simulink model "simulator_LQR"  (R2018b)
settings: Solver=VariableStepAuto  StartTime=0.0  StopTime=150  RelTol=1e-5
values from neighbouring files (symbols this model uses):
  C = [1 0 0;0 1 0; 0 0 1]    [parameters_LQR.m]
  LQR_fast = [830.7,	3032.2,	1268.5]    [parameters_LQR.m]
  LQR_slow = [624.5,	2682.3,	1569.3]    [parameters_LQR.m]
  Nbar = Nu + [(LQR_slow(2)+LQR_fast(2))/2 (LQR_slow(3)+LQR_fast(3))/2]*Nx    [parameters_LQR.m]
undefined symbols (not defined in the file or in its folder): A, B
libraries: simulink_extras x2
settings Model: Creator=jenny  LastModifiedBy=jenny

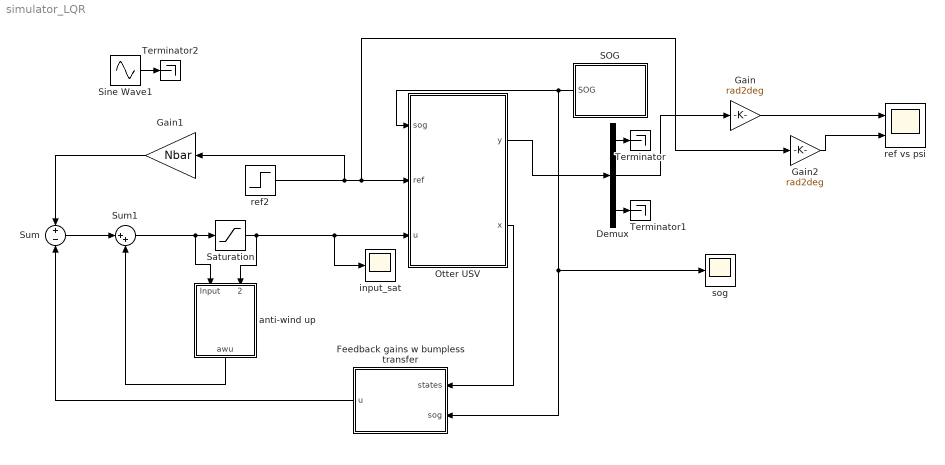
== system simulator_LQR ==
  Demux : Demux  Outputs=3
  Feedback gains w bumpless transfer : Subsystem
  Gain : Gain  Gain=rad2deg
  Gain1 : Gain  Gain=Nbar
  Gain2 : Gain  Gain=rad2deg
  Otter USV : Subsystem
  SOG : Subsystem
  Saturation : Saturate  UpperLimit=73.6  LowerLimit=-73.6
  Sine Wave1 : Sin  Amplitude=pi/6  Frequency=0.05  SampleTime=0
  Sum : Sum  Inputs=+|-
  Sum1 : Sum  Inputs=|++
  Terminator : Terminator
  Terminator1 : Terminator
  Terminator2 : Terminator
  anti-wind up : Subsystem
  input_sat : Scope
  ref vs psi : Scope  NumInputPorts=2
  ref2 : Step  Time=0  After=pi/6  SampleTime=0
  sog : Scope
  wires:
  SOG/1(SOG) -> Otter USV/1(sog), Feedback gains w bumpless transfer/2(sog), sog/1
  Otter USV/2(x) -> Feedback gains w bumpless transfer/1(states)
  ref2/1 -> Gain2/1, Otter USV/2(ref), Gain1/1
  Saturation/1 -> input_sat/1, Otter USV/3(u), anti-wind up/2(Input sat)
  Sum/1 -> Sum1/1
  Sum1/1 -> anti-wind up/1(Input), Saturation/1
  anti-wind up/1(awu) -> Sum1/2
  Feedback gains w bumpless transfer/1(u) -> Sum/2
  Gain1/1 -> Sum/1
  Otter USV/1(y) -> Demux/1
  Gain/1 -> ref vs psi/1
  Gain2/1 -> ref vs psi/2
  Demux/2 -> Gain/1
  Demux/1 -> Terminator/1
  Demux/3 -> Terminator1/1
  Sine Wave1/1 -> Terminator2/1

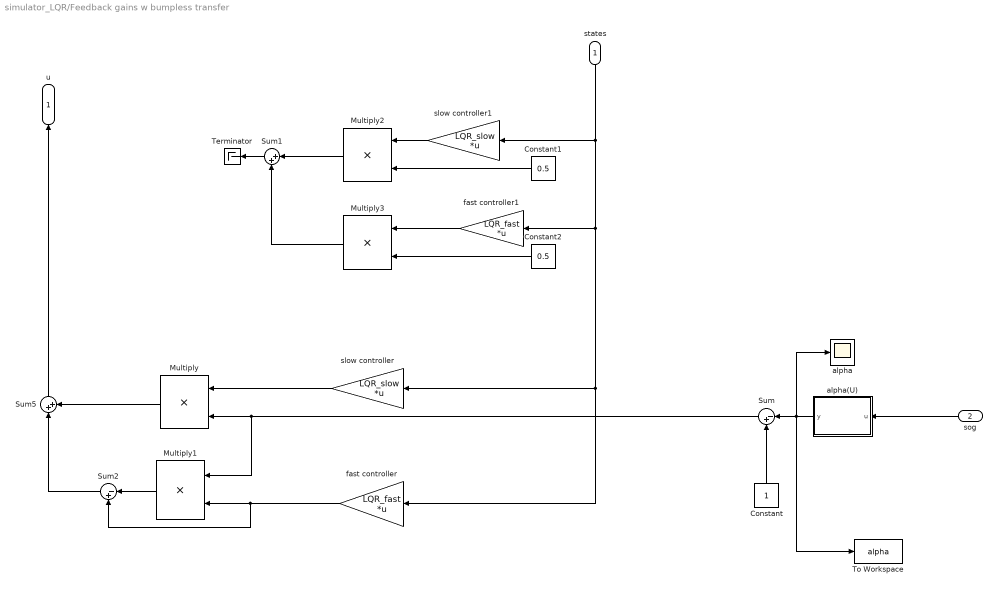
== system simulator_LQR/Feedback gains w bumpless transfer ==
  states : Inport
  sog : Inport  Port=2
  Constant : Constant
  Constant1 : Constant  Value=0.5
  Constant2 : Constant  Value=0.5
  Multiply{,1..3} (4 alike) : Product
  Sum : Sum  Inputs=|-+
  Sum1 : Sum  Inputs=|++
  Sum2 : Sum  Inputs=|-+
  Sum5 : Sum  Inputs=|++
  Terminator : Terminator
  To Workspace : ToWorkspace  VariableName=alpha  SampleTime=-1
  alpha : Scope
  alpha(U) : MATLAB Function  TreatAsAtomicUnit=on
  fast controller : Gain  Gain=LQR_fast  Multiplication=Matrix(K*u)
  fast controller1 : Gain  Gain=LQR_fast  Multiplication=Matrix(K*u)
  slow controller : Gain  Gain=LQR_slow  Multiplication=Matrix(K*u)
  slow controller1 : Gain  Gain=LQR_slow  Multiplication=Matrix(K*u)
  u : Outport
  wires:
  Constant/1 -> Sum/2
  alpha(U)/1(y) -> To Workspace/1, alpha/1, Sum/1
  fast controller/1 -> Sum2/2, Multiply1/2
  slow controller/1 -> Multiply/1
  Multiply1/1 -> Sum2/1
  sog/1 -> alpha(U)/1(u)
  Sum/1 -> Multiply1/1, Multiply/2
  Sum2/1 -> Sum5/1
  Multiply/1 -> Sum5/2
  slow controller1/1 -> Multiply2/1
  Constant1/1 -> Multiply2/2
  Multiply2/1 -> Sum1/1
  fast controller1/1 -> Multiply3/1
  Multiply3/1 -> Sum1/2
  Constant2/1 -> Multiply3/2
  states/1 -> slow controller1/1, fast controller/1, slow controller/1, fast controller1/1
  Sum5/1 -> u/1
  Sum1/1 -> Terminator/1

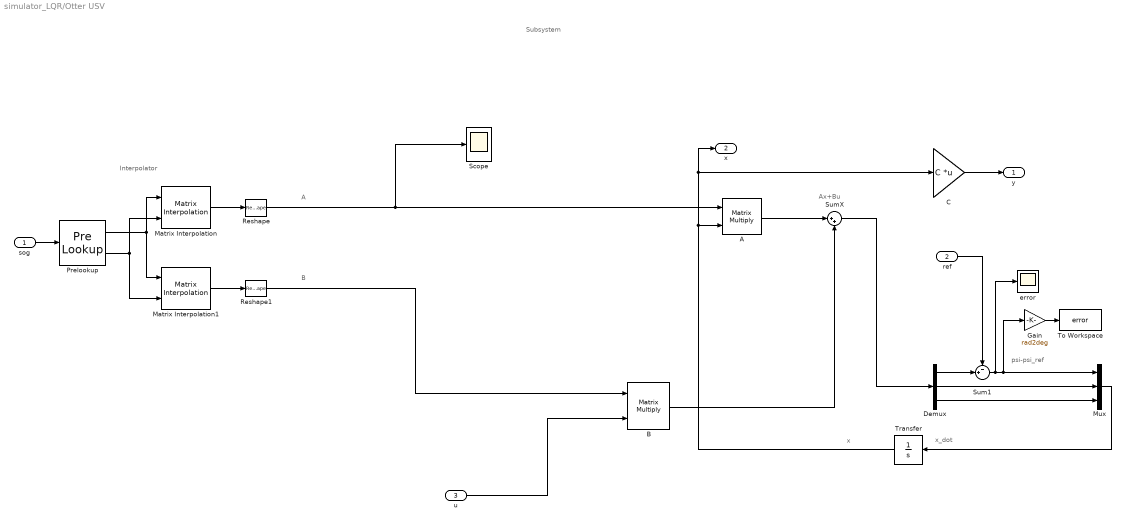
== system simulator_LQR/Otter USV ==
  note: A
  note: Interpolator
  note: Ax+Bu
  note: x_dot
  note: x
  note: psi-psi_ref
  note: Subsystem
  note: B
  sog : Inport
  ref : Inport  Port=2
  u : Inport  Port=3
  A : Product  Multiplication=Matrix(*)
  B : Product  Multiplication=Matrix(*)
  C : Gain  Gain=C  Multiplication=Matrix(K*u)  SaturateOnIntegerOverflow=on  OutDataTypeStr=Inherit: Same as input  ParamDataTypeStr=Inherit: Same as input
  Demux : Demux  Outputs=3
  Gain : Gain  Gain=rad2deg
  Matrix Interpolation : simulink_extras/Additional Lookup Tables/Matrix Interpolation  InterpMethod=Linear  ExtrapMethod=Clip  InterpolateDimension=1  TableData=A  SimulateUsing=Code generation
      settings: SourceProductName=Simulink  SourceProductBaseCode=SL
  Matrix Interpolation1 : simulink_extras/Additional Lookup Tables/Matrix Interpolation  InterpMethod=Linear  ExtrapMethod=Clip  InterpolateDimension=1  TableData=B  SimulateUsing=Code generation
      settings: SourceProductName=Simulink  SourceProductBaseCode=SL
  Mux : Mux  Inputs=3
  Prelookup : PreLookup  BreakpointsData=0:0.5:2  ExtrapMethod=Linear
  Reshape : Reshape  OutputDimensionality=Customize  OutputDimensions=[3,3]
  Reshape1 : Reshape  OutputDimensionality=Column vector (2-D)
  Scope : Scope
  Sum1 : Sum  Inputs=-+|
  SumX : Sum  Inputs=|++  SaturateOnIntegerOverflow=on  InputSameDT=on  OutDataTypeStr=Inherit: Same as first input
  To Workspace : ToWorkspace  VariableName=error  SampleTime=-1
  Transfer : Integrator
  error : Scope
  y : Outport
  x : Outport  Port=2
  wires:
  Mux/1 -> Transfer/1
  C/1 -> y/1
  sog/1 -> Prelookup/1
  B/1 -> SumX/2
  Sum1/1 -> error/1, Gain/1, Mux/1
  Demux/3 -> Mux/3
  SumX/1 -> Demux/1
  Reshape/1 -> Scope/1, A/1
  u/1 -> B/2
  Reshape1/1 -> B/1
  A/1 -> SumX/1
  Demux/2 -> Mux/2
  Transfer/1 -> x/1, C/1, A/2
  ref/1 -> Sum1/1
  Prelookup/2 -> Matrix Interpolation/2, Matrix Interpolation1/2
  Prelookup/1 -> Matrix Interpolation/1, Matrix Interpolation1/1
  Matrix Interpolation1/1 -> Reshape1/1
  Matrix Interpolation/1 -> Reshape/1
  Gain/1 -> To Workspace/1
  Demux/1 -> Sum1/2

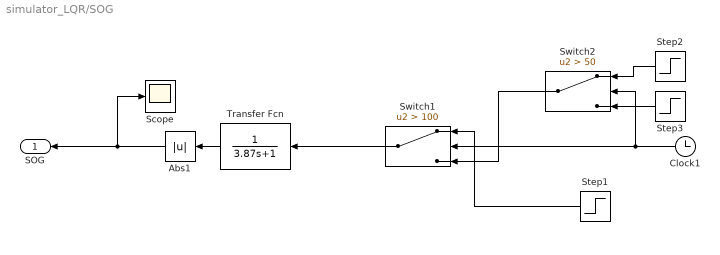
== system simulator_LQR/SOG ==
  Abs1 : Abs
  Clock1 : Clock
  Scope : Scope
  Step1 : Step  Time=0  After=0.5  SampleTime=0
  Step2 : Step  Time=0  After=2  SampleTime=0
  Step3 : Step  Time=0  After=0.3  SampleTime=0
  Switch1 : Switch  Criteria=u2 > Threshold  Threshold=100
  Switch2 : Switch  Criteria=u2 > Threshold  Threshold=50
  Transfer Fcn : TransferFcn  Denominator=[3.87 1]
  SOG : Outport
  wires:
  Transfer Fcn/1 -> Abs1/1
  Abs1/1 -> Scope/1, SOG/1
  Clock1/1 -> Switch2/2, Switch1/2
  Switch1/1 -> Transfer Fcn/1
  Step2/1 -> Switch2/1
  Step3/1 -> Switch2/3
  Switch2/1 -> Switch1/3
  Step1/1 -> Switch1/1

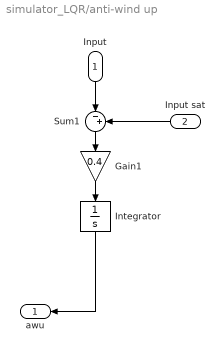
== system simulator_LQR/anti-wind up ==
  Input : Inport
  Input sat : Inport  Port=2
  Gain1 : Gain  Gain=0.4
  Integrator : Integrator
  Sum1 : Sum  Inputs=|-+
  awu : Outport
  wires:
  Gain1/1 -> Integrator/1
  Input/1 -> Sum1/1
  Sum1/1 -> Gain1/1
  Input sat/1 -> Sum1/2
  Integrator/1 -> awu/1

== matlab function simulator_LQR/Feedback gains w bumpless transfer/alpha(U) ==
  data: u input; y output
function y = fcn(u)
% Max speed of otter with sonar is 2 m/s
    max_speed = 2;
    u_norm = min(u/max_speed,1);        % Normalizing the speed
    
    fast_ex = 4;                       % Tuneable exponent. Small values give steeper slope 

    fast_b = (0.5-0.5^fast_ex)/(1-0.5^fast_ex); 
    
    
    if u_norm >= 0 && u_norm <= .3 
        alpha = min(u_norm,0.3);
    elseif u_norm > .3 && u_norm < .5
        alpha = min(u_norm,0.5);
    else
        %alpha = min(u_norm,1);
        alpha = min((1-fast_b)*u_norm^fast_ex + fast_b,1);
    end

y = alpha;
